simulink model "AntiWindup_FF"  (R2021a)
settings: Solver=ode45  StartTime=0.0  StopTime=8  RelTol=1e-3
undefined symbols (not defined in the file): drv, est_par, gbox, K_w, kd_best, ki_best, kp_best, mot, rads2rpm, rpm2degs, sens, simp_model
libraries: simulink x2
settings Model: Creator=Utente  LastModifiedBy=gioel
settings SolverCC: ZeroCrossAlgorithm=Adaptive  AlgebraicLoopSolver=TrustRegion
settings DataIOCC: SaveFormat=StructureWithTime  ReturnWorkspaceOutputs=off
settings DebuggingCC: IgnoredZcDiagnostic=none  SFMachineParentedDataDiag=warning

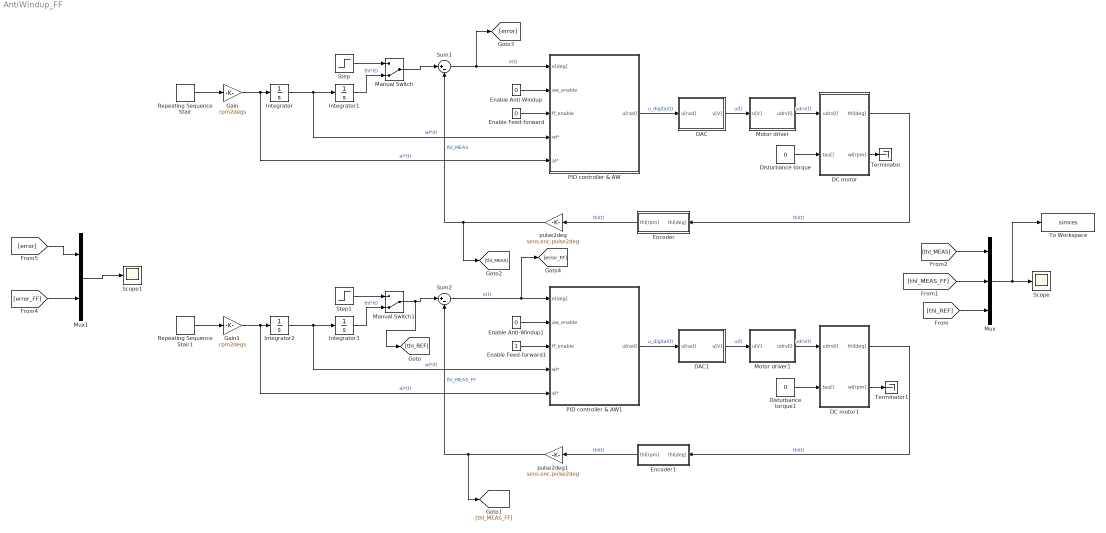
== system AntiWindup_FF ==
  DAC : Subsystem
  DAC1 : Subsystem
  DC motor : Subsystem
  DC motor1 : Subsystem
  Disturbance torque : Constant  Value=0
  Disturbance torque1 : Constant  Value=0
  Enable Anti-Windup : Constant  Value=0
  Enable Anti-Windup1 : Constant  Value=0
  Enable Feed-forward : Constant  Value=0
  Enable Feed-forward1 : Constant
  Encoder : Subsystem
  Encoder1 : Subsystem
  Gain : Gain  Gain=rpm2degs
  Gain1 : Gain  Gain=rpm2degs
  Integrator{,1..3} (4 alike) : Integrator
  Manual Switch : ManualSwitch  CurrentSetting=0
  Manual Switch1 : ManualSwitch  CurrentSetting=0
  Motor driver : Subsystem
  Motor driver1 : Subsystem
  Mux : Mux  Inputs=3
  Mux1 : Mux  Inputs=2
  PID controller & AW : Subsystem
  PID controller & AW1 : Subsystem
  Repeating Sequence Stair : simulink/Sources/Repeating Sequence Stair  OutValues=[900 0 -900 -900 0 900].'  tsamp=0.5  OutMin=[]  OutMax=[]  OutDataTypeStr=double  OutputDataTypeScalingMode=double  OutDataType=fixdt(0,8)  ConRadixGroup=Best Precision: Vector-wise  OutScaling=2^-12
  Repeating Sequence Stair1 : simulink/Sources/Repeating Sequence Stair  OutValues=[900 0 -900 -900 0 900].'  tsamp=0.5  OutMin=[]  OutMax=[]  OutDataTypeStr=double  OutputDataTypeScalingMode=double  OutDataType=fixdt(0,8)  ConRadixGroup=Best Precision: Vector-wise  OutScaling=2^-12
  Scope : Scope
  Scope1 : Scope
  Step : Step  Time=0  After=360  SampleTime=0
  Step1 : Step  Time=0  After=360  SampleTime=0
  Sum1 : Sum  Inputs=|+-
  Sum2 : Sum  Inputs=|+-
  Terminator : Terminator
  Terminator1 : Terminator
  To Workspace : ToWorkspace  VariableName=simres  SaveFormat=Structure With Time  SampleTime=-1
  pulse2deg : Gain  Gain=sens.enc.pulse2deg
  pulse2deg1 : Gain  Gain=sens.enc.pulse2deg
  wires:
  Motor driver/1(udrv[I]) -> DC motor/1(udrv[I])  "udrv(t)"
  DAC/1(u[V]) -> Motor driver/1(u[V])  "u(t)"
  Encoder/1(thl[rpm]) -> pulse2deg/1  "thl(t)"
  pulse2deg/1 -> [thl_MEAS], Sum1/2  "thl_MEAS"
  Sum1/1 -> [error], PID controller & AW/1(e[deg])  "e(t)"
  PID controller & AW/1(u[rad]) -> DAC/1(u[rad])  "u_digital(t)"
  DC motor/1(thl[deg]) -> Encoder/1(thl[deg])  "thl(t)"
  Step/1 -> Manual Switch/1
  Disturbance torque/1 -> DC motor/2(tau[])
  Enable Anti-Windup/1 -> PID controller & AW/2(aw_enable)
  Manual Switch/1 -> Sum1/1
  Enable Feed-forward/1 -> PID controller & AW/3(ff_enable)
  Repeating Sequence Stair/1 -> Gain/1
  Gain/1 -> PID controller & AW/5(al*), Integrator/1  "al*(t)"
  Integrator1/1 -> Manual Switch/2  "thl*(t)"
  Integrator/1 -> Integrator1/1, PID controller & AW/4(wl*)  "wl*(t)"
  Integrator2/1 -> PID controller & AW1/4(wl*), Integrator3/1  "wl*(t)"
  Integrator3/1 -> Manual Switch1/2  "thl*(t)"
  Gain1/1 -> Integrator2/1, PID controller & AW1/5(al*)  "al*(t)"
  Repeating Sequence Stair1/1 -> Gain1/1
  Enable Feed-forward1/1 -> PID controller & AW1/3(ff_enable)
  Manual Switch1/1 -> [thl_REF], Sum2/1
  Enable Anti-Windup1/1 -> PID controller & AW1/2(aw_enable)
  Disturbance torque1/1 -> DC motor1/2(tau[])
  Step1/1 -> Manual Switch1/1
  DC motor1/1(thl[deg]) -> Encoder1/1(thl[deg])  "thl(t)"
  PID controller & AW1/1(u[rad]) -> DAC1/1(u[rad])  "u_digital(t)"
  Sum2/1 -> [error_FF], PID controller & AW1/1(e[deg])  "e(t)"
  pulse2deg1/1 -> [thl_MEAS_FF], Sum2/2  "thl_MEAS_FF"
  Encoder1/1(thl[rpm]) -> pulse2deg1/1  "thl(t)"
  DAC1/1(u[V]) -> Motor driver1/1(u[V])  "u(t)"
  Motor driver1/1(udrv[I]) -> DC motor1/1(udrv[I])  "udrv(t)"
  Mux/1 -> To Workspace/1, Scope/1
  [thl_MEAS] -> Mux/1
  [error] -> Mux1/1
  [error_FF] -> Mux1/2
  Mux1/1 -> Scope1/1
  DC motor/2(wl[rpm]) -> Terminator/1
  DC motor1/2(wl[rpm]) -> Terminator1/1
  [thl_MEAS_FF] -> Mux/2
  [thl_REF] -> Mux/3

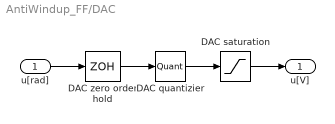
== system AntiWindup_FF/DAC ==
  u[rad] : Inport
  DAC quantizier : Quantizer  QuantizationInterval=daq.dac.q
  DAC saturation : Saturate  UpperLimit=10  LowerLimit=-10
  DAC zero order hold : ZeroOrderHold  SampleTime=sens.enc.T_s
  u[V] : Outport
  wires:
  DAC quantizier/1 -> DAC saturation/1
  DAC zero order hold/1 -> DAC quantizier/1
  DAC saturation/1 -> u[V]/1
  u[rad]/1 -> DAC zero order hold/1

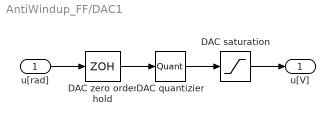
== system AntiWindup_FF/DAC1 ==
  u[rad] : Inport
  DAC quantizier : Quantizer  QuantizationInterval=daq.dac.q
  DAC saturation : Saturate  UpperLimit=10  LowerLimit=-10
  DAC zero order hold : ZeroOrderHold  SampleTime=sens.enc.T_s
  u[V] : Outport
  wires:
  u[rad]/1 -> DAC zero order hold/1
  DAC saturation/1 -> u[V]/1
  DAC zero order hold/1 -> DAC quantizier/1
  DAC quantizier/1 -> DAC saturation/1

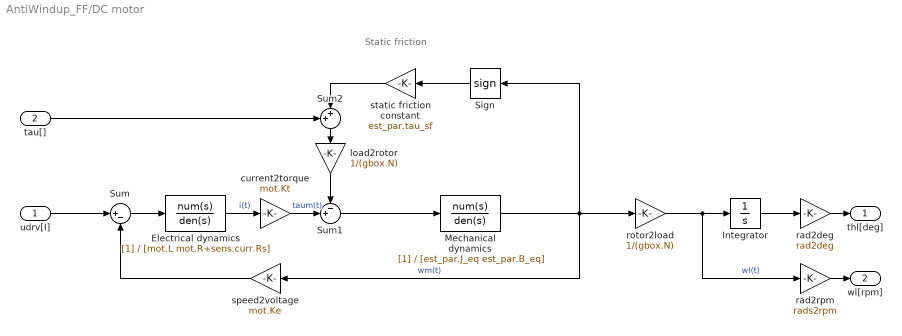
== system AntiWindup_FF/DC motor ==
  note: Static friction
  udrv[I] : Inport  Unit=V
  tau[] : Inport  Port=2  Unit=V
  Electrical dynamics : TransferFcn  Denominator=[mot.L mot.R+sens.curr.Rs]
  Integrator : Integrator
  Mechanical dynamics : TransferFcn  Denominator=[est_par.J_eq est_par.B_eq]
  Sign : Signum  ZeroCross=off
  Sum : Sum  Inputs=|+-
  Sum1 : Sum  Inputs=-+|
  Sum2 : Sum  Inputs=++|
  current2torque : Gain  Gain=mot.Kt
  load2rotor : Gain  Gain=1/(gbox.N)
  rad2deg : Gain  Gain=rad2deg
  rad2rpm : Gain  Gain=rads2rpm
  rotor2load : Gain  Gain=1/(gbox.N)
  speed2voltage : Gain  Gain=mot.Ke
  static friction constant : Gain  Gain=est_par.tau_sf
  thl[deg] : Outport  Unit=deg
  wl[rpm] : Outport  Port=2  Unit=rpm
  wires:
  load2rotor/1 -> Sum1/1
  Mechanical dynamics/1 -> Sign/1, rotor2load/1, speed2voltage/1  "wm(t)"
  Sign/1 -> static friction constant/1
  current2torque/1 -> Sum1/2  "taum(t)"
  Sum1/1 -> Mechanical dynamics/1
  speed2voltage/1 -> Sum/2
  rotor2load/1 -> rad2rpm/1, Integrator/1  "wl(t)"
  Electrical dynamics/1 -> current2torque/1  "i(t)"
  Integrator/1 -> rad2deg/1
  Sum/1 -> Electrical dynamics/1
  rad2rpm/1 -> wl[rpm]/1
  rad2deg/1 -> thl[deg]/1
  udrv[I]/1 -> Sum/1
  static friction constant/1 -> Sum2/2
  Sum2/1 -> load2rotor/1
  tau[]/1 -> Sum2/1

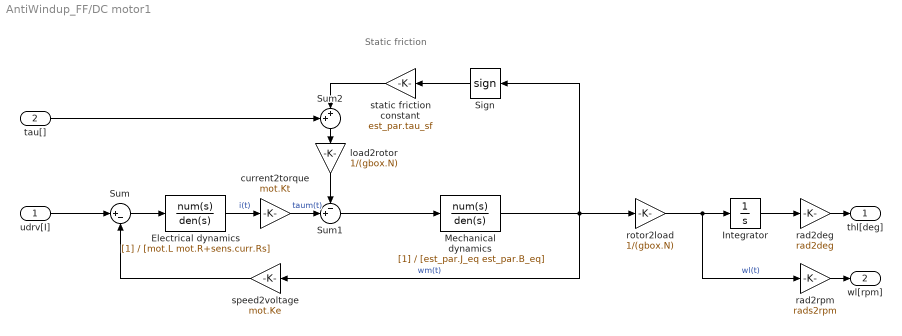
== system AntiWindup_FF/DC motor1 ==
  note: Static friction
  udrv[I] : Inport  Unit=V
  tau[] : Inport  Port=2  Unit=V
  Electrical dynamics : TransferFcn  Denominator=[mot.L mot.R+sens.curr.Rs]
  Integrator : Integrator
  Mechanical dynamics : TransferFcn  Denominator=[est_par.J_eq est_par.B_eq]
  Sign : Signum  ZeroCross=off
  Sum : Sum  Inputs=|+-
  Sum1 : Sum  Inputs=-+|
  Sum2 : Sum  Inputs=++|
  current2torque : Gain  Gain=mot.Kt
  load2rotor : Gain  Gain=1/(gbox.N)
  rad2deg : Gain  Gain=rad2deg
  rad2rpm : Gain  Gain=rads2rpm
  rotor2load : Gain  Gain=1/(gbox.N)
  speed2voltage : Gain  Gain=mot.Ke
  static friction constant : Gain  Gain=est_par.tau_sf
  thl[deg] : Outport  Unit=deg
  wl[rpm] : Outport  Port=2  Unit=rpm
  wires:
  tau[]/1 -> Sum2/1
  Sum2/1 -> load2rotor/1
  static friction constant/1 -> Sum2/2
  udrv[I]/1 -> Sum/1
  rad2deg/1 -> thl[deg]/1
  rad2rpm/1 -> wl[rpm]/1
  Sum/1 -> Electrical dynamics/1
  Integrator/1 -> rad2deg/1
  Electrical dynamics/1 -> current2torque/1  "i(t)"
  rotor2load/1 -> Integrator/1, rad2rpm/1  "wl(t)"
  speed2voltage/1 -> Sum/2
  Sum1/1 -> Mechanical dynamics/1
  current2torque/1 -> Sum1/2  "taum(t)"
  Sign/1 -> static friction constant/1
  Mechanical dynamics/1 -> speed2voltage/1, rotor2load/1, Sign/1  "wm(t)"
  load2rotor/1 -> Sum1/1

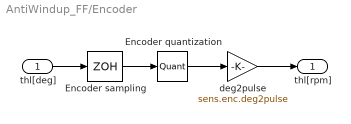
== system AntiWindup_FF/Encoder ==
  thl[deg] : Inport
  Encoder quantization : Quantizer  QuantizationInterval=sens.enc.q
  Encoder sampling : ZeroOrderHold  SampleTime=0.001
  deg2pulse : Gain  Gain=sens.enc.deg2pulse
  thl[rpm] : Outport
  wires:
  Encoder quantization/1 -> deg2pulse/1
  deg2pulse/1 -> thl[rpm]/1
  Encoder sampling/1 -> Encoder quantization/1
  thl[deg]/1 -> Encoder sampling/1

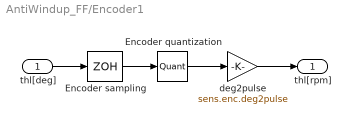
== system AntiWindup_FF/Encoder1 ==
  thl[deg] : Inport
  Encoder quantization : Quantizer  QuantizationInterval=sens.enc.q
  Encoder sampling : ZeroOrderHold  SampleTime=0.001
  deg2pulse : Gain  Gain=sens.enc.deg2pulse
  thl[rpm] : Outport
  wires:
  thl[deg]/1 -> Encoder sampling/1
  Encoder sampling/1 -> Encoder quantization/1
  deg2pulse/1 -> thl[rpm]/1
  Encoder quantization/1 -> deg2pulse/1

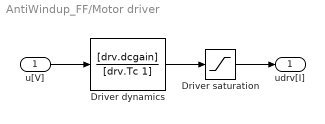
== system AntiWindup_FF/Motor driver ==
  u[V] : Inport
  Driver dynamics : TransferFcn  Numerator=[drv.dcgain]  Denominator=[drv.Tc 1]
  Driver saturation : Saturate  UpperLimit=12  LowerLimit=-12
  udrv[I] : Outport
  wires:
  Driver saturation/1 -> udrv[I]/1
  Driver dynamics/1 -> Driver saturation/1
  u[V]/1 -> Driver dynamics/1

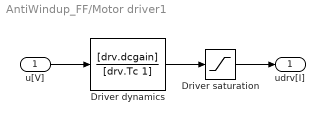
== system AntiWindup_FF/Motor driver1 ==
  u[V] : Inport
  Driver dynamics : TransferFcn  Numerator=[drv.dcgain]  Denominator=[drv.Tc 1]
  Driver saturation : Saturate  UpperLimit=12  LowerLimit=-12
  udrv[I] : Outport
  wires:
  u[V]/1 -> Driver dynamics/1
  Driver dynamics/1 -> Driver saturation/1
  Driver saturation/1 -> udrv[I]/1

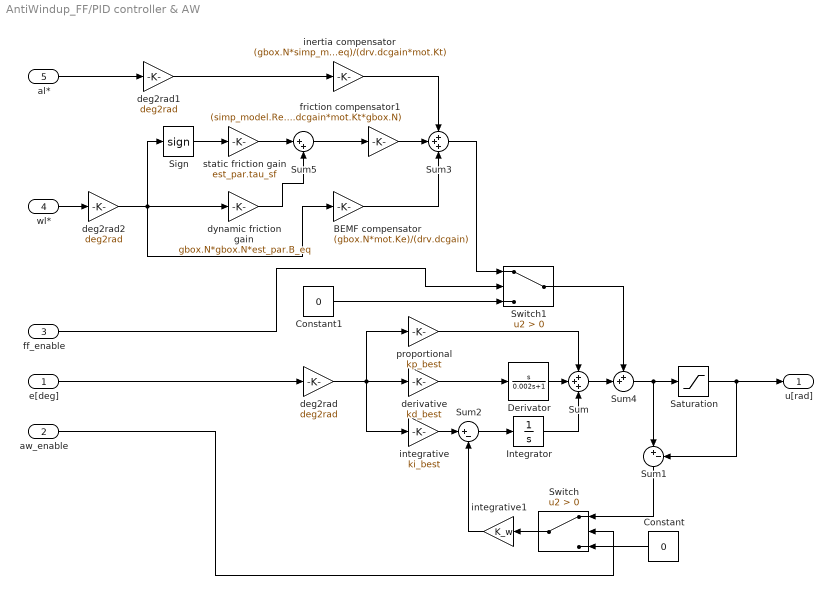
== system AntiWindup_FF/PID controller & AW ==
  e[deg] : Inport  Unit=deg
  aw_enable : Inport  Port=2  Unit=deg
  ff_enable : Inport  Port=3  Unit=deg
  wl* : Inport  Port=4  Unit=deg
  al* : Inport  Port=5  Unit=deg
  BEMF compensator : Gain  Gain=(gbox.N*mot.Ke)/(drv.dcgain)
  Constant : Constant  Value=0
  Constant1 : Constant  Value=0
  Derivator : TransferFcn  Numerator=[1 0]  Denominator=[0.002 1]
  Integrator : Integrator
  Saturation : Saturate  UpperLimit=10  LowerLimit=-10
  Sign : Signum
  Sum : Sum  Inputs=+++
  Sum1 : Sum  Inputs=|+-
  Sum2 : Sum  Inputs=|+-
  Sum3 : Sum  Inputs=+++
  Sum4 : Sum  Inputs=++|
  Sum5 : Sum  Inputs=|++
  Switch : Switch  Criteria=u2 > Threshold
  Switch1 : Switch  Criteria=u2 > Threshold
  deg2rad : Gain  Gain=deg2rad
  deg2rad1 : Gain  Gain=deg2rad
  deg2rad2 : Gain  Gain=deg2rad
  derivative : Gain  Gain=kd_best
  dynamic friction gain : Gain  Gain=gbox.N*gbox.N*est_par.B_eq
  friction compensator1 : Gain  Gain=(simp_model.Req)/(drv.dcgain*mot.Kt*gbox.N)
  inertia compensator : Gain  Gain=(gbox.N*simp_model.Req*est_par.J_eq)/(drv.dcgain*mot.Kt)
  integrative : Gain  Gain=ki_best
  integrative1 : Gain  Gain=K_w
  proportional : Gain  Gain=kp_best
  static friction gain : Gain  Gain=est_par.tau_sf
  u[rad] : Outport
  wires:
  e[deg]/1 -> deg2rad/1
  deg2rad/1 -> integrative/1, derivative/1, proportional/1
  proportional/1 -> Sum/1
  Saturation/1 -> Sum1/2, u[rad]/1
  integrative/1 -> Sum2/1
  Sum2/1 -> Integrator/1
  integrative1/1 -> Sum2/2
  Integrator/1 -> Sum/3
  Derivator/1 -> Sum/2
  derivative/1 -> Derivator/1
  aw_enable/1 -> Switch/2
  Constant/1 -> Switch/3
  Switch/1 -> integrative1/1
  Sum1/1 -> Switch/1
  ff_enable/1 -> Switch1/2
  Constant1/1 -> Switch1/3
  friction compensator1/1 -> Sum3/2
  inertia compensator/1 -> Sum3/1
  BEMF compensator/1 -> Sum3/3
  Sum4/1 -> Sum1/1, Saturation/1
  Switch1/1 -> Sum4/1
  Sign/1 -> static friction gain/1
  static friction gain/1 -> Sum5/1
  dynamic friction gain/1 -> Sum5/2
  Sum5/1 -> friction compensator1/1
  al*/1 -> deg2rad1/1
  wl*/1 -> deg2rad2/1
  Sum3/1 -> Switch1/1
  Sum/1 -> Sum4/2
  deg2rad1/1 -> inertia compensator/1
  deg2rad2/1 -> BEMF compensator/1, Sign/1, dynamic friction gain/1

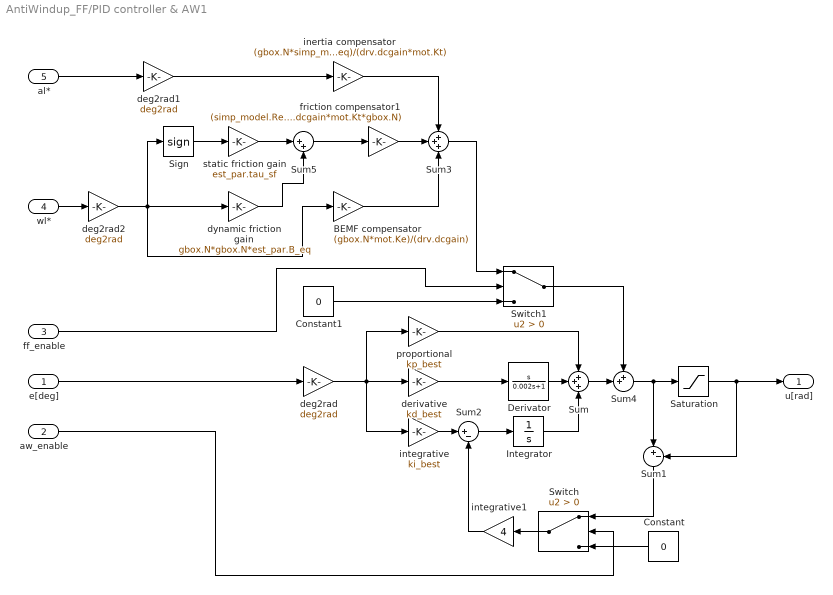
== system AntiWindup_FF/PID controller & AW1 ==
  e[deg] : Inport  Unit=deg
  aw_enable : Inport  Port=2  Unit=deg
  ff_enable : Inport  Port=3  Unit=deg
  wl* : Inport  Port=4  Unit=deg
  al* : Inport  Port=5  Unit=deg
  BEMF compensator : Gain  Gain=(gbox.N*mot.Ke)/(drv.dcgain)
  Constant : Constant  Value=0
  Constant1 : Constant  Value=0
  Derivator : TransferFcn  Numerator=[1 0]  Denominator=[0.002 1]
  Integrator : Integrator
  Saturation : Saturate  UpperLimit=10  LowerLimit=-10
  Sign : Signum
  Sum : Sum  Inputs=+++
  Sum1 : Sum  Inputs=|+-
  Sum2 : Sum  Inputs=|+-
  Sum3 : Sum  Inputs=+++
  Sum4 : Sum  Inputs=++|
  Sum5 : Sum  Inputs=|++
  Switch : Switch  Criteria=u2 > Threshold
  Switch1 : Switch  Criteria=u2 > Threshold
  deg2rad : Gain  Gain=deg2rad
  deg2rad1 : Gain  Gain=deg2rad
  deg2rad2 : Gain  Gain=deg2rad
  derivative : Gain  Gain=kd_best
  dynamic friction gain : Gain  Gain=gbox.N*gbox.N*est_par.B_eq
  friction compensator1 : Gain  Gain=(simp_model.Req)/(drv.dcgain*mot.Kt*gbox.N)
  inertia compensator : Gain  Gain=(gbox.N*simp_model.Req*est_par.J_eq)/(drv.dcgain*mot.Kt)
  integrative : Gain  Gain=ki_best
  integrative1 : Gain  Gain=4
  proportional : Gain  Gain=kp_best
  static friction gain : Gain  Gain=est_par.tau_sf
  u[rad] : Outport
  wires:
  deg2rad2/1 -> dynamic friction gain/1, Sign/1, BEMF compensator/1
  deg2rad1/1 -> inertia compensator/1
  Sum/1 -> Sum4/2
  Sum3/1 -> Switch1/1
  wl*/1 -> deg2rad2/1
  al*/1 -> deg2rad1/1
  Sum5/1 -> friction compensator1/1
  dynamic friction gain/1 -> Sum5/2
  static friction gain/1 -> Sum5/1
  Sign/1 -> static friction gain/1
  Switch1/1 -> Sum4/1
  Sum4/1 -> Saturation/1, Sum1/1
  BEMF compensator/1 -> Sum3/3
  inertia compensator/1 -> Sum3/1
  friction compensator1/1 -> Sum3/2
  Constant1/1 -> Switch1/3
  ff_enable/1 -> Switch1/2
  Sum1/1 -> Switch/1
  Switch/1 -> integrative1/1
  Constant/1 -> Switch/3
  aw_enable/1 -> Switch/2
  derivative/1 -> Derivator/1
  Derivator/1 -> Sum/2
  Integrator/1 -> Sum/3
  integrative1/1 -> Sum2/2
  Sum2/1 -> Integrator/1
  integrative/1 -> Sum2/1
  Saturation/1 -> u[rad]/1, Sum1/2
  proportional/1 -> Sum/1
  deg2rad/1 -> proportional/1, derivative/1, integrative/1
  e[deg]/1 -> deg2rad/1
